simulink model "PCM_System"  (R2021a)
settings: Solver=VariableStepAuto  StartTime=0.0  StopTime=5  MaxStep=0.00001  RelTol=1e-3
values from neighbouring files (symbols this model uses):
  fs = 15000    [FIRMaker.m]    (also in IIR_code.m = 48000)
  hzDen = [1 zeros(1,(length(hzNum)-1))]    [FIRMaker.m]
  hzNum = zeros(1,tap)    [FIRMaker.m]
libraries: dspsrcs4 x1, dspsigops x1
settings Model: Creator=james  LastModifiedBy=jroutley

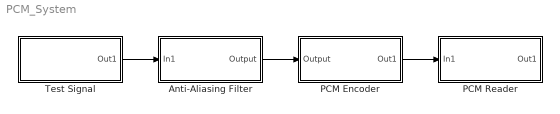
== system PCM_System ==
  Anti-Aliasing Filter : Subsystem
  PCM Encoder : Subsystem
  PCM Reader : Subsystem
  Test Signal : Subsystem
  wires:
  PCM Encoder/1(Out1) -> PCM Reader/1(In1)
  Test Signal/1(Out1) -> Anti-Aliasing Filter/1(In1)
  Anti-Aliasing Filter/1(Output) -> PCM Encoder/1(Output)

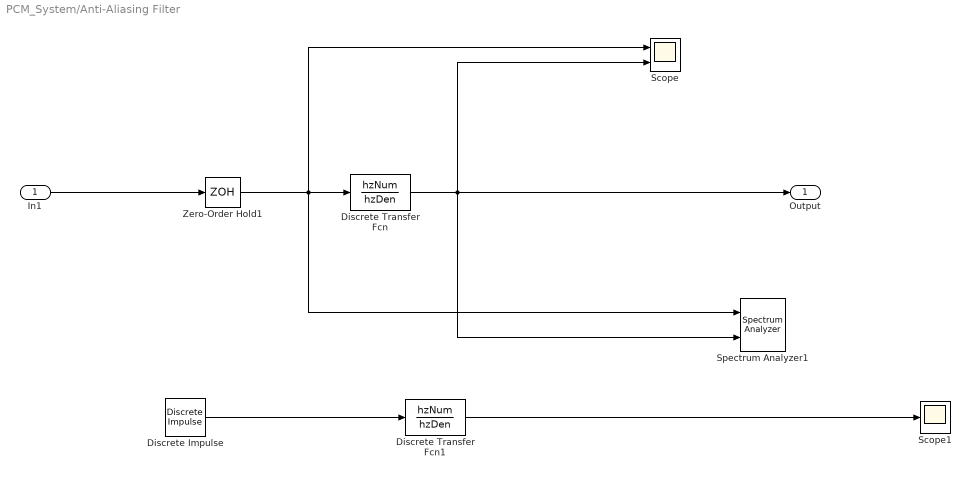
== system PCM_System/Anti-Aliasing Filter ==
  In1 : Inport
  Discrete Transfer Fcn : DiscreteTransferFcn  Numerator=hzNum  Denominator=hzDen
  Discrete Transfer Fcn1 : DiscreteTransferFcn  Numerator=hzNum  Denominator=hzDen
  Discrete Impulse : dspsrcs4/Discrete  Impulse  Delay=0  SampleTime=0.001  FrameSample=1  OutputFrames=off  dataType=double  isSigned=on  wordLen=16  udDataType=sfix(16)  fracBitsMode=Best precision  numFracBits=15  OutDataTypeStr=double  LastOutDataTypeStr=double
  Scope : Scope  NumInputPorts=2
  Scope1 : Scope
  Spectrum Analyzer1 : SpectrumAnalyzer  NumInputPorts=2
  Zero-Order Hold1 : ZeroOrderHold  SampleTime=1/fs
  Output : Outport
  wires:
  Discrete Transfer Fcn/1 -> Spectrum Analyzer1/2, Scope/2, Output/1
  Zero-Order Hold1/1 -> Spectrum Analyzer1/1, Scope/1, Discrete Transfer Fcn/1
  In1/1 -> Zero-Order Hold1/1
  Discrete Impulse/1 -> Discrete Transfer Fcn1/1
  Discrete Transfer Fcn1/1 -> Scope1/1

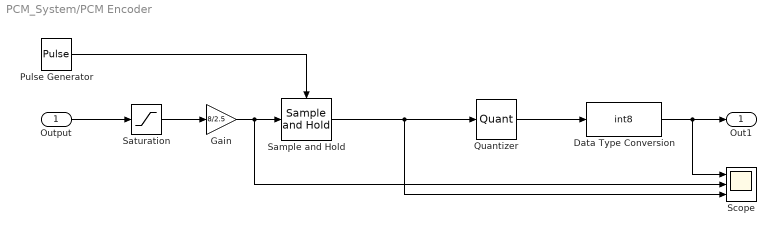
== system PCM_System/PCM Encoder ==
  Output : Inport
  Data Type Conversion : DataTypeConversion  OutDataTypeStr=int8
  Gain : Gain  Gain=8/2.5
  Pulse Generator : DiscretePulseGenerator  PulseType=Time based  Period=0.1  PulseWidth=5
  Quantizer : Quantizer  QuantizationInterval=1  LinearizeAsGain=off
  Sample and Hold : dspsigops/Sample and Hold  trig=Rising edge  initCond=0  latchinput=off
  Saturation : Saturate  UpperLimit=2.5  LowerLimit=-2.5
  Scope : Scope  NumInputPorts=3
  Out1 : Outport
  wires:
  Data Type Conversion/1 -> Scope/1, Out1/1
  Quantizer/1 -> Data Type Conversion/1
  Output/1 -> Saturation/1
  Saturation/1 -> Gain/1
  Sample and Hold/1 -> Scope/3, Quantizer/1
  Gain/1 -> Scope/2, Sample and Hold/1
  Pulse Generator/1 -> Sample and Hold/Trigger

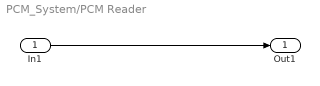
== system PCM_System/PCM Reader ==
  In1 : Inport
  Out1 : Outport
  wires:
  In1/1 -> Out1/1

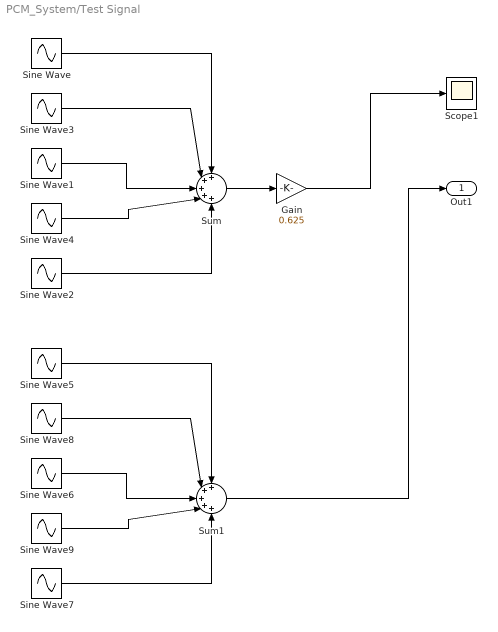
== system PCM_System/Test Signal ==
  Gain : Gain  Gain=0.625
  Scope1 : Scope
  Sine Wave : Sin  Frequency=1300*2*pi  SampleTime=0
  Sine Wave1 : Sin  Frequency=3200*2*pi  SampleTime=0
  Sine Wave2 : Sin  Frequency=6300*2*pi  SampleTime=0
  Sine Wave3 : Sin  Frequency=2400*2*pi  SampleTime=0
  Sine Wave4 : Sin  Frequency=5600*2*pi  SampleTime=0
  Sine Wave5 : Sin  Frequency=6000*2*pi  SampleTime=0
  Sine Wave6 : Sin  Frequency=6400*2*pi  SampleTime=0
  Sine Wave7 : Sin  Frequency=6800*2*pi  SampleTime=0
  Sine Wave8 : Sin  Frequency=6200*2*pi  SampleTime=0
  Sine Wave9 : Sin  Frequency=6600*2*pi  SampleTime=0
  Sum : Sum  Inputs=+++++
  Sum1 : Sum  Inputs=+++++
  Out1 : Outport
  wires:
  Sine Wave1/1 -> Sum/3
  Gain/1 -> Scope1/1
  Sine Wave3/1 -> Sum/2
  Sine Wave/1 -> Sum/1
  Sum/1 -> Gain/1
  Sine Wave4/1 -> Sum/4
  Sine Wave2/1 -> Sum/5
  Sine Wave8/1 -> Sum1/2
  Sine Wave7/1 -> Sum1/5
  Sine Wave6/1 -> Sum1/3
  Sine Wave9/1 -> Sum1/4
  Sine Wave5/1 -> Sum1/1
  Sum1/1 -> Out1/1
